simulink model "STM32_Nucleo_Programming"  (R2023a)
settings: Solver=FixedStepDiscrete  StartTime=0.0  StopTime=inf  FixedStep=0.01  RelTol=1e-3  EnableMultiTasking=on
libraries: mbedblockslib x2, stm32blockslib x2
settings Model: SimulationMode=external  ExtModeTrigDuration=10  Creator=JesseJabezArendse  LastModifiedBy=JesseJabezArendse
settings OptimizationCC: EnhancedBackFolding=on  PassReuseOutputArgsAs=Individual arguments  ZeroExternalMemoryAtStartup=off  ZeroInternalMemoryAtStartup=off  MaxStackSize=64  OptimizeBlockOrder=speed  DifferentSizesBufferReuse=on  OptimizationCustomize=off  EfficientTunableParamExpr=on
settings DebuggingCC: ParameterPrecisionLossMsg=none  ParameterTunabilityLossMsg=error
settings HardwareCC: ProdBitPerPointer=32  ProdBitPerSizeT=32  ProdBitPerPtrDiffT=32  ProdLargestAtomicInteger=Long  ProdLargestAtomicFloat=Double  ProdWordSize=32  ProdLongLongMode=on  ProdHWDeviceType=ARM Compatible->ARM Cortex
settings SFSimCC: MATLABDynamicMemAlloc=off
settings RTWCC: Description=Embedded Coder  SystemTargetFile=ert.tlc  HardwareBoard=STM32 Nucleo F411RE  TemplateMakefile=ert_default_tmf  Toolchain=GNU Tools for ARM Embedded Processors  BuildConfiguration=Specify
settings RTWCC: CustomHeaderCode=|
  | #include "NucleoMX\Core\Inc\CustomDump.h"
  | #include "NucleoMX\Core\Inc\usart.h"
  | #include "NucleoMX\Core\Inc\main.h"
settings RTWCC: CustomInclude=|
  | NucleoMX\Core\Inc\
  | NucleoMX\Core\Src\
settings RTWCC: CustomSource=|
  | NucleoMX\Core\Src\CustomDump.c
  | NucleoMX\Core\Src\usart.c
  | NucleoMX\Core\Src\main.c
settings CodeAppCC: ForceParamTrailComments=on  IgnoreCustomStorageClasses=off  OperatorAnnotations=on  SimulinkDataObjDesc=on  SFDataObjDesc=on  InsertBlockDesc=on
settings ERTTargetCC: CodeReplacementLibrary=ARM Cortex-M  SupportContinuousTime=on  ExtModeTransport=3  ExtModeStaticAlloc=on  ExtModeStaticAllocSize=2000  ExtModeMexFile=ext_xcp  ExtModeIntrfLevel=Level2 - Open

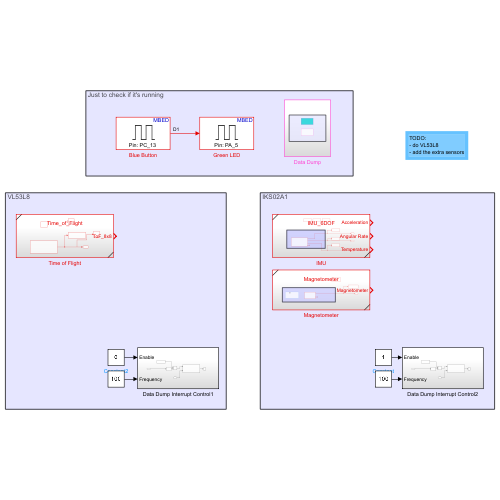
[thumbnail: Simulink's stored preview of the top-level diagram]
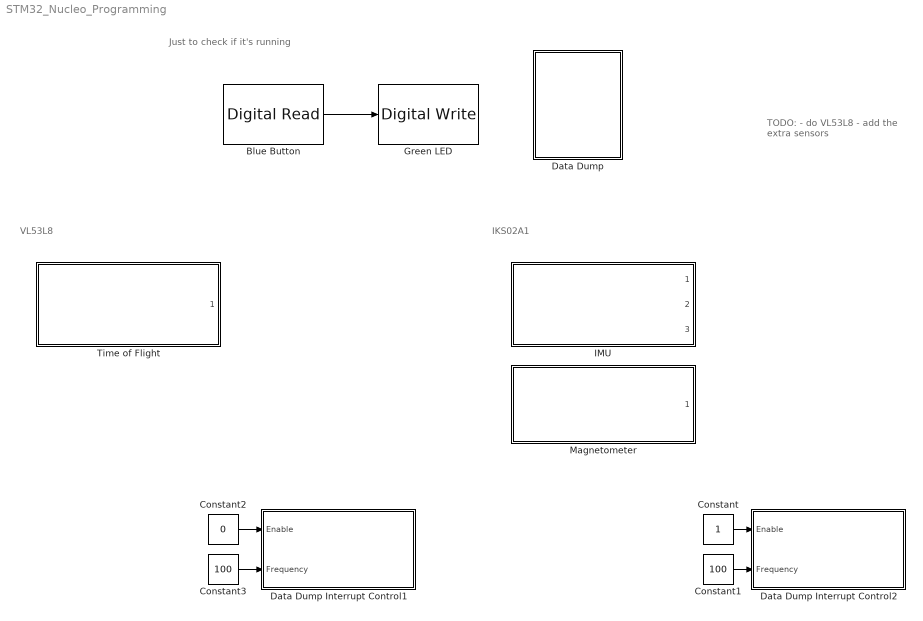
== system STM32_Nucleo_Programming ==
  note: TODO:
      | - do VL53L8
      | - add the extra sensors
  note: Just to check if it's running
  note: IKS02A1
  note: VL53L8
  Blue Button : mbedblockslib/Digital Read  Pin=PC_13  Direction=input  SampleTime=-1
      settings: LibrarySourceBlock=stmnucleorootlib/Common/Digital Read
  Constant : Constant
  Constant1 : Constant  Value=100
  Constant2 : Constant  Value=0
  Constant3 : Constant  Value=100
  Data Dump : Subsystem
  Data Dump Interrupt Control1 : Subsystem
  Data Dump Interrupt Control2 : Subsystem
  Green LED : mbedblockslib/Digital Write  Pin=PA_5  Direction=output
      settings: LibrarySourceBlock=stmnucleorootlib/Common/Digital Write
  IMU : Subsystem  ReferencedSubsystem=IMU_6DOF
  Magnetometer : Subsystem  ReferencedSubsystem=Magnetometer
  Time of Flight : Subsystem  ReferencedSubsystem=Time_of_Flight
  wires:
  Blue Button/1 -> Green LED/1
  Constant/1 -> Data Dump Interrupt Control2/1(Enable)
  Constant1/1 -> Data Dump Interrupt Control2/2(Frequency)
  Constant2/1 -> Data Dump Interrupt Control1/1(Enable)
  Constant3/1 -> Data Dump Interrupt Control1/2(Frequency)

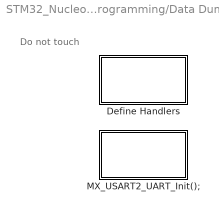
== system STM32_Nucleo_Programming/Data Dump ==
  note: Do not touch
  Define Handlers : Subsystem  mask(Model Source){ShowInLibBrowser=0}
      mask prompts: ShowInLibBrowser "Simulink:masks:CustCodeMaskParam1_MP"
      settings: CopyFcn=cccopyfcn(gcb)  OpenFcn=ccopenfcn('Model Source')
      mask Help: eval('feval(''rtwprivate'',''rtwhelpview'',''rtw_model_source_block'')');
      mask Display: disp('Model\nSource');
  MX_USART2_UART_Init(); : Subsystem  mask(System Initialize){ShowInLibBrowser=0}
      mask prompts: ShowInLibBrowser "Simulink:masks:CustCodeMaskParam1_MP"
      settings: CopyFcn=cccopyfcn(gcb)  OpenFcn=ccopenfcn('System Initialize Function')
      mask Help: eval('feval(''rtwprivate'',''rtwhelpview'',''rtw_sys_initialize_block'')');
      mask Display: disp('System\nInitialize');

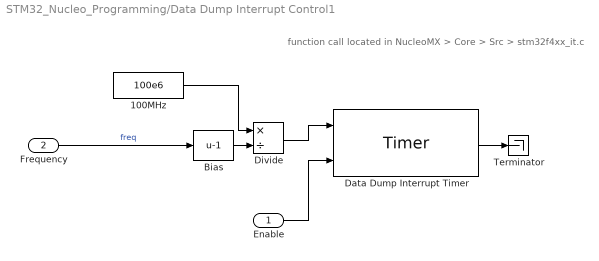
== system STM32_Nucleo_Programming/Data Dump Interrupt Control1 ==
  note: function call located in NucleoMX > Core > Src > stm32f4xx_it.c
  Enable : Inport
  Frequency : Inport  Port=2
  100MHz : Constant  Value=100e6
  Bias : Bias  Bias=-1  SaturateOnIntegerOverflow=off
  Data Dump Interrupt Timer : stm32blockslib/Timer  Priority=4  TimerModule=TIM3  EnableFrequencyInput=on  EnableCounterInput=on  EnableMainOutputInput=off  SetRCAfterCE=off  OutputDirection=off  OutputMainOutputEnableStatus=off  SampleTime=-1  EnableUpdateEvent=off  EnableCaptureCompare1Event=off  EnableCaptureCompare2Event=off  EnableCaptureCompare3Event=off  EnableCaptureCompare4Event=off  EnableTriggerEvent=off  EnableBreakEvent=off  EnableBreakEvent2=off  EnableCOMGenerationEvent=off  ProcessorFamily=STM32F7
      settings: LibrarySourceBlock=stm32f4xxblockslib/Timer
  Divide : Product  Inputs=*/
  Terminator : Terminator
  wires:
  Divide/1 -> Data Dump Interrupt Timer/1
  Frequency/1 -> Bias/1  "freq"
  Data Dump Interrupt Timer/1 -> Terminator/1
  100MHz/1 -> Divide/1
  Bias/1 -> Divide/2
  Enable/1 -> Data Dump Interrupt Timer/2

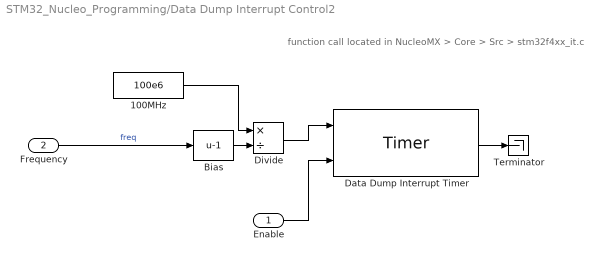
== system STM32_Nucleo_Programming/Data Dump Interrupt Control2 ==
  note: function call located in NucleoMX > Core > Src > stm32f4xx_it.c
  Enable : Inport
  Frequency : Inport  Port=2
  100MHz : Constant  Value=100e6
  Bias : Bias  Bias=-1  SaturateOnIntegerOverflow=off
  Data Dump Interrupt Timer : stm32blockslib/Timer  Priority=4  TimerModule=TIM2  EnableFrequencyInput=on  EnableCounterInput=on  EnableMainOutputInput=off  SetRCAfterCE=off  OutputDirection=off  OutputMainOutputEnableStatus=off  SampleTime=-1  EnableUpdateEvent=off  EnableCaptureCompare1Event=off  EnableCaptureCompare2Event=off  EnableCaptureCompare3Event=off  EnableCaptureCompare4Event=off  EnableTriggerEvent=off  EnableBreakEvent=off  EnableBreakEvent2=off  EnableCOMGenerationEvent=off  ProcessorFamily=STM32F7
      settings: LibrarySourceBlock=stm32f4xxblockslib/Timer
  Divide : Product  Inputs=*/
  Terminator : Terminator
  wires:
  Divide/1 -> Data Dump Interrupt Timer/1
  Frequency/1 -> Bias/1  "freq"
  Data Dump Interrupt Timer/1 -> Terminator/1
  100MHz/1 -> Divide/1
  Bias/1 -> Divide/2
  Enable/1 -> Data Dump Interrupt Timer/2

== system STM32_Nucleo_Programming/Data Dump/Define Handlers ==

== system STM32_Nucleo_Programming/Data Dump/MX_USART2_UART_Init(); ==
